simulink model "multi_sensor_with_filtering"  (R2018b)
settings: Solver=FixedStepAuto  StartTime=0.0  StopTime=inf  RelTol=1e-3  EnableMultiTasking=on
model workspace (MAT data in the model file):
  sensorControlMatrix = [0  0  0; 0  0  0; 0  0  0; 0  0  0; 0  0  0; 0  0  0; 1  0  0; 0  1  0; 0  0  1; 0  0  0; 0  0  0; 0  0  0; 0  0  0; 0  0  0; 0  0  0]
  sensorProcessNoiseMatrix = [1  0  0  0.02  0  0  0.0002  0  0  0  0  0  0  0  0; 0  1  0  0  0.02  0  0  0.0002  0  0  0  0  0  0  0; 0  0  1  0  0  0.02  0  0  0.0002  0  0  0  0  0  0; 0.02  0  0  1  0  0  0.02  0  0  0  0  0  0  0  0; 0  0.02  0  0  1  0  0  0.02  0  0  0  0  0  0  0; 0  0  0.02  0  0  1  0  0  0.02  0  0  0  0  0  0; 0.0002  0  0  0.02  0  0  1  0  0  0  0  0  0  0  0; 0  0.0002  0  0  0.02  0  0  1  0  0  0  0  0  0  0; 0  0  0.0002  0  0  0.02  0  0  1  0  0  0  0  0  0; 0  0  0  0  0  0  0  0  0  1  0  0  0.02  0  0; 0  0  0  0  0  0  0  0  0  0  1  0  0  0.02  0; 0  0  0  0  0  0  0  0  0  0  0  1  0  0  0.02; 0  0  0  0  0  0  0  0  0  0.02  0  0  1  0  0; 0  0  0  0  0  0  0  0  0  0  0.02  0  0  1  0; 0  0  0  0  0  0  0  0  0  0  0  0.02  0  0  1]
  sensorSampleTime = 0.01
  sensorSystemMatrix = [1  0  0  0.02  0  0  0.0002  0  0  0  0  0  0  0  0; 0  1  0  0  0.02  0  0  0.0002  0  0  0  0  0  0  0; 0  0  1  0  0  0.02  0  0  0.0002  0  0  0  0  0  0; 0  0  0  1  0  0  0.02  0  0  0  0  0  0  0  0; 0  0  0  0  1  0  0  0.02  0  0  0  0  0  0  0; 0  0  0  0  0  1  0  0  0.02  0  0  0  0  0  0; 0  0  0  0  0  0  1  0  0  0  0  0  0  0  0; 0  0  0  0  0  0  0  1  0  0  0  0  0  0  0; 0  0  0  0  0  0  0  0  1  0  0  0  0  0  0; 0  0  0  0  0  0  0  0  0  1  0  0  0.02  0  0; 0  0  0  0  0  0  0  0  0  0  1  0  0  0.02  0; 0  0  0  0  0  0  0  0  0  0  0  1  0  0  0.02; 0  0  0  0  0  0  0  0  0  0  0  0  1  0  0; 0  0  0  0  0  0  0  0  0  0  0  0  0  1  0; 0  0  0  0  0  0  0  0  0  0  0  0  0  0  1]
undefined symbols (not defined in the file): DiscIntNeverNeededParam, q
libraries: dspfdesign x5, sharedtransform x4, sharedTrackingLibrary x2, aerolibutil x2, simulink_extras x2, pil_lib x1
settings Model: SimulationMode=accelerator  ExtModeTrigDuration=2  Creator=Aliak  LastModifiedBy=Aliak
settings OptimizationCC: EnhancedBackFolding=on  PassReuseOutputArgsAs=Individual arguments  EfficientMapNaN2IntZero=off  MaxStackSize=64  OptimizeBlockOrder=speed  DifferentSizesBufferReuse=on  OptimizationCustomize=off
settings DebuggingCC: ParameterTunabilityLossMsg=error
settings HardwareCC: ProdBitPerInt=16  ProdBitPerPointer=16  ProdBitPerSizeT=16  ProdBitPerPtrDiffT=16  ProdWordSize=8  ProdHWDeviceType=Atmel->AVR  TargetBitPerPointer=64  TargetBitPerSizeT=64  TargetBitPerPtrDiffT=64  TargetLongLongMode=on  TargetIntDivRoundTo=Zero  TargetEndianess=LittleEndian  TargetWordSize=64  TargetHWDeviceType=MATLAB Host
settings SFSimCC: MATLABDynamicMemAlloc=off
settings RTWCC: SystemTargetFile=ert.tlc  HardwareBoard=Arduino Uno  TemplateMakefile=ert_default_tmf  GenerateReport=on  Toolchain=Arduino AVR  BuildConfiguration=Faster Runs  IncludeHyperlinkInReport=on  LaunchReport=on  CreateSILPILBlock=PIL  GenerateTraceInfo=on  GenerateTraceReport=on  GenerateTraceReportSl=on  GenerateTraceReportSf=on  GenerateTraceReportEml=on
settings CodeAppCC: ForceParamTrailComments=on  IgnoreCustomStorageClasses=off  MaxIdLength=128  OperatorAnnotations=on  SimulinkDataObjDesc=on  SFDataObjDesc=on  InsertBlockDesc=on
settings ERTTargetCC: SupportContinuousTime=on  SupportVariableSizeSignals=on

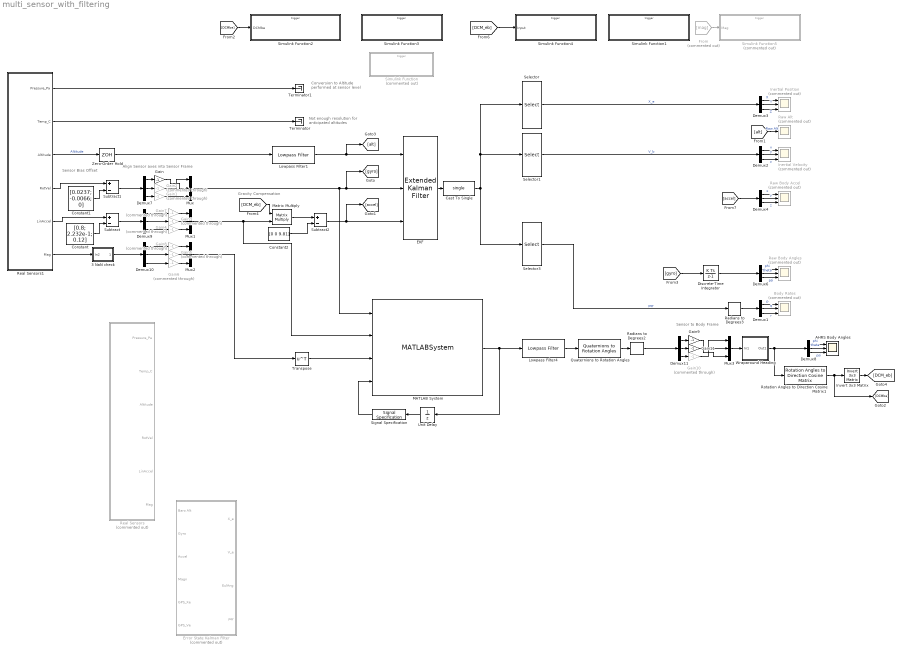
== system multi_sensor_with_filtering ==
  note: Sensor Bias Offset
  note: Gravity Compensation
  note: Align Sensor axes into Sensor Frame
  note: Sensor to Body Frame
  note: Conversion to Altitude performed at sensor level
  note: Not enough resolution for anticipated altitudes
  3 NaN check : Subsystem
  AHRS Body Angles : Scope  NumInputPorts=3
  Body Rates : Scope  Commented=on  NumInputPorts=3
  Cast To Single : DataTypeConversion  OutDataTypeStr=single
  Constant : Constant  Value=[0.8; 2.232e-1; 0.12]  VectorParams1D=off
  Constant1 : Constant  Value=[0.0237; -0.0066; 0]  VectorParams1D=off
  Constant2 : Constant  Value=[0 0 9.81]
  Demux{1..4,6..11} (10 alike) : Demux  Outputs=3
  Discrete-Time Integrator : DiscreteIntegrator  SampleTime=-1  ICPrevOutput=DiscIntNeverNeededParam  ICPrevScaledInput=DiscIntNeverNeededParam
  EKF : sharedTrackingLibrary/Extended Kalman Filter  StateTransitionFcn=sensorStateTransitionFcn  HasStateTransitionJacobianFcn=off  StateTransitionJacobianFcn=identityJacobianFcn  HasAdditiveProcessNoise=Additive  ProcessNoise=0.02  HasTimeVaryingProcessNoise=off  HasStateTransitionFcnExtraArgument=0  InitialState=single([0;0;49;0;0;0;0;0;0;0;0;0;0;0;0;])  InitialStateCovariance=0.0001  MeasurementFcn1=altMeasurementFcn  HasMeasurementJacobianFcn1=off  MeasurementJacobianFcn1=identityJacobianFcn  HasMeasurementEnablePort1=off  HasAdditiveMeasurementNoise1=Additive  MeasurementNoise1=0.18  HasTimeVaryingMeasurementNoise1=off  HasMeasurementFcnExtraArgument1=0  MeasurementFcn2=gyroMeasurementFcn  HasMeasurementJacobianFcn2=off  MeasurementJacobianFcn2=identityJacobianFcn  HasMeasurementEnablePort2=off  HasAdditiveMeasurementNoise2=Additive  MeasurementNoise2=0.1*eye(3)  HasTimeVaryingMeasurementNoise2=off  HasMeasurementFcnExtraArgument2=0  MeasurementFcn3=accelMeasurementFcn  HasMeasurementJacobianFcn3=off  MeasurementJacobianFcn3=identityJacobianFcn  HasMeasurementEnablePort3=off  HasAdditiveMeasurementNoise3=Additive  MeasurementNoise3=0.016*eye(3)  HasTimeVaryingMeasurementNoise3=off  HasMeasurementFcnExtraArgument3=0  MeasurementFcn4=magMeasurementFcn  HasMeasurementJacobianFcn4=off  MeasurementJacobianFcn4=identityJacobianFcn  HasMeasurementEnablePort4=off  HasAdditiveMeasurementNoise4=Additive  MeasurementNoise4=5*eye(3)  HasTimeVaryingMeasurementNoise4=off  HasMeasurementFcnExtraArgument4=0  MeasurementFcn5=myMeasurementFcn  HasMeasurementJacobianFcn5=off  HasMeasurementEnablePort5=off  HasAdditiveMeasurementNoise5=Additive  MeasurementNoise5=1  HasTimeVaryingMeasurementNoise5=off  HasMeasurementFcnExtraArgument5=0  EnableMultirate=off  StateTransitionFcnSampleTime=1  MeasurementFcn1SampleTime=1  MeasurementFcn2SampleTime=1  MeasurementFcn3SampleTime=1  MeasurementFcn4SampleTime=1  MeasurementFcn5SampleTime=1  UseCurrentEstimator=on  OutputStateCovariance=off  DataType=single  SampleTime=sensorSampleTime  NumberOfMeasurements=3
      settings: SourceProductName=Control System Toolbox  SourceProductBaseCode=CT
  Error State Kalman FIlter : Subsystem  Commented=on
  From : From  Commented=on  GotoTag=mag
  Gain : Gain  Gain=-1
  Gain{1..4,7,10} (6 alike) : Gain  Commented=through  Gain=-1
  Gain11 : Gain  Gain=-1
  Gain5 : Gain  Commented=through  Gain=-1  OutDataTypeStr=single
  Gain6 : Gain  Commented=through  Gain=-1  OutDataTypeStr=single
  Gain8 : Gain  Commented=through  Gain=-1  OutDataTypeStr=single
  Gain9 : Gain  Gain=-1
  Inertial Position : Scope  Commented=on  NumInputPorts=3
  Inertial Velocity : Scope  Commented=on  NumInputPorts=3
  Invert 3x3 Matrix : aerolibutil/Invert  3x3 Matrix
  Lowpass Filter1 : dspfdesign/Lowpass Filter  FilterType=IIR  DesignForMinimumOrder=on  FilterOrder=50  PassbandFrequency=250  StopbandFrequency=500  PassbandRipple=0.1  StopbandAttenuation=80  InheritSampleRate=off  SampleRate=1100  SimulateUsing=Code generation  roundingMode=Floor  coeffsDataTypeStr=fixdt(1,16)
  Lowpass Filter4 : dspfdesign/Lowpass Filter  FilterType=FIR  DesignForMinimumOrder=on  FilterOrder=50  PassbandFrequency=200  StopbandFrequency=300  PassbandRipple=0.1  StopbandAttenuation=80  InheritSampleRate=off  SampleRate=700  SimulateUsing=Code generation  roundingMode=Floor  coeffsDataTypeStr=fixdt(1,16)
  MATLAB System : MATLABSystem  System=MadgwickAHRSFilter  SamplePeriod=sensorSampleTime  Beta=5  SimulateUsing=Code generation
      mask Type: MadgwickAHRSFilter
      mask Display:
      | disp('MadgwickAHRSFilter');
      | port_label('input',1,'Gyroscope');
      | port_label('input',2,'Accelerometer');
      | port_label('input',3,'Magnetometer');
      | port_label('input',4,'q');
      | port_label('output',1,'quat');
  Matrix Multiply : Product  Multiplication=Matrix(*)
  Mux{,1..3} (4 alike) : Mux  Inputs=3
  Quaternions to Rotation Angles : sharedtransform/Quaternions to Rotation Angles  rotationOrder=ZYX  aMode=aMode
      settings: SourceProductBaseCode=AE
  Radians to Degrees2 : simulink_extras/Transformations/Radians to Degrees
  Radians to Degrees3 : simulink_extras/Transformations/Radians to Degrees
  Raw Alt : Scope  Commented=on
  Raw Body Accel : Scope  Commented=on  NumInputPorts=3
  Raw Body Angles : Scope  Commented=on  NumInputPorts=3
  Real Sensors : Subsystem  Commented=on  VariantControl=SimType==1
  Real Sensors1 : Subsystem  DialogController=pil_create_dialog  LoadFcn=|
      | try
      |    if ~strcmp(rtw.pil.getPILVersion, '9.5 (R2018b)_13')
      |       set_param(gcb, 'DialogController', '');
      |       set_param(gcb, 'DialogControllerArgs', '');
      |    end
      | catch e
      |       set_param(gcb, 'DialogController', '');
      |       set_param(gcb, 'DialogControllerArgs', '');
      | end
      mask help: PIL:pil:XILBlockMaskDesc
      mask Display: disp('PIL');
  Rotation Angles to Direction Cosine Matrix1 : sharedtransform/Rotation Angles to Direction Cosine Matrix  rotationOrder=XYZ  aMode=aMode
      settings: SourceProductBaseCode=AE
  Selector : Selector  IndexMode=Zero-based  InputPortWidth=15  IndexOptions=Index vector (dialog)  Indices=[0 1 2]  OutputSizes=1
  Selector1 : Selector  IndexMode=Zero-based  InputPortWidth=15  IndexOptions=Index vector (dialog)  Indices=[3 4 5]  OutputSizes=1
  Selector3 : Selector  IndexMode=Zero-based  InputPortWidth=15  IndexOptions=Index vector (dialog)  Indices=[12 13 14]  OutputSizes=1
  Signal Specification : SignalSpecification  OutDataTypeStr=single  Dimensions=[1 4]
  Simulink Function : Subsystem  Commented=on  TreatAsAtomicUnit=on
  Simulink Function1 : Subsystem  TreatAsAtomicUnit=on
  Simulink Function2 : Subsystem  TreatAsAtomicUnit=on
  Simulink Function3 : Subsystem  TreatAsAtomicUnit=on
  Simulink Function4 : Subsystem  TreatAsAtomicUnit=on
  Simulink Function5 : Subsystem  Commented=on  TreatAsAtomicUnit=on
  Subtract : Sum  Inputs=+-  OutDataTypeStr=single
  Subtract1 : Sum  Inputs=+-  OutDataTypeStr=single
  Subtract2 : Sum  Inputs=+-  OutDataTypeStr=single
  Terminator : Terminator
  Terminator1 : Terminator
  Transpose : Math  Operator=transpose  SaturateOnIntegerOverflow=on
  Unit Delay : UnitDelay  InitialCondition=[1 0 0 0]  SampleTime=sensorSampleTime
  Wraparound Heading : Subsystem
  Zero-Order Hold : ZeroOrderHold  SampleTime=sensorSampleTime
  wires:
  Selector3/1 -> Radians to Degrees3/1  "pqr"
  Cast To Single/1 -> Selector/1, Selector1/1, Selector3/1
  From/1 -> Simulink Function5/1(Mag)
  Subtract/1 -> Demux9/1
  EKF/1 -> Cast To Single/1
  [DCMbe] -> Simulink Function2/1(DCMbe)
  Selector/1 -> Demux3/1  "X_e"
  Selector1/1 -> Demux2/1  "V_b"
  Radians to Degrees3/1 -> Demux1/1
  Demux1/1 -> Body Rates/1  "p"
  Demux1/2 -> Body Rates/2  "q"
  Demux1/3 -> Body Rates/3  "r"
  Demux2/1 -> Inertial Velocity/1  "x"
  Demux2/2 -> Inertial Velocity/2  "y"
  Demux2/3 -> Inertial Velocity/3  "z"
  Demux3/1 -> Inertial Position/1  "X"
  Demux3/2 -> Inertial Position/2  "Y"
  Demux3/3 -> Inertial Position/3  "Z"
  [accel] -> Demux4/1
  Demux4/2 -> Raw Body Accel/2  "y"
  Demux4/1 -> Raw Body Accel/1  "x"
  Demux4/3 -> Raw Body Accel/3  "z"
  Constant/1 -> Subtract/2
  Constant1/1 -> Subtract1/2
  [alt] -> Raw Alt/1  "Raw Alt"
  Demux6/3 -> Raw Body Angles/3  "psi"
  Demux6/1 -> Raw Body Angles/1  "phi"
  Demux6/2 -> Raw Body Angles/2  "theta"
  [gyro] -> Discrete-Time Integrator/1
  Discrete-Time Integrator/1 -> Demux6/1
  Subtract1/1 -> Demux7/1
  Demux8/3 -> AHRS Body Angles/3  "psi"
  Demux8/2 -> AHRS Body Angles/2  "theta"
  Quaternions to Rotation Angles/1 -> Radians to Degrees2/1
  Demux8/1 -> AHRS Body Angles/1  "phi"
  Transpose/1 -> MATLAB System/3
  Lowpass Filter1/1 -> EKF/1, [alt]
  Mux/1 -> EKF/2, [gyro], MATLAB System/1
  Zero-Order Hold/1 -> Lowpass Filter1/1
  Real Sensors1/2(Temp_C) -> Terminator/1
  Real Sensors1/3(Altitude) -> Zero-Order Hold/1  "Altitude"
  Real Sensors1/5(LinAccel) -> Subtract/1
  Real Sensors1/1(Pressure_Pa) -> Terminator1/1
  Mux2/1 -> Transpose/1
  Real Sensors1/4(RotVel) -> Subtract1/1
  [DCM_eb] -> Matrix Multiply/1
  Subtract2/1 -> [accel], EKF/3
  [DCM_eb] -> Simulink Function4/1(Input)
  Invert 3x3 Matrix/1 -> [DCM_eb]
  Rotation Angles to Direction Cosine Matrix1/1 -> [DCMbe], Invert 3x3 Matrix/1
  Matrix Multiply/1 -> Subtract2/1
  Constant2/1 -> Subtract2/2
  Unit Delay/1 -> Signal Specification/1
  MATLAB System/1 -> Lowpass Filter4/1, Unit Delay/1
  Signal Specification/1 -> MATLAB System/4
  Mux1/1 -> MATLAB System/2, Matrix Multiply/2
  Real Sensors1/6(Mag) -> 3 NaN check/1(In2)
  3 NaN check/1(Out1) -> Demux10/1
  Lowpass Filter4/1 -> Quaternions to Rotation Angles/1
  Demux10/3 -> Gain6/1
  Demux10/1 -> Gain8/1
  Demux10/2 -> Gain5/1
  Demux9/3 -> Gain4/1
  Demux9/2 -> Gain3/1
  Demux9/1 -> Gain7/1
  Demux7/3 -> Gain1/1
  Demux7/1 -> Gain/1
  Demux7/2 -> Gain2/1
  Gain3/1 -> Mux1/2
  Gain4/1 -> Mux1/3
  Gain5/1 -> Mux2/2
  Gain6/1 -> Mux2/3
  Gain7/1 -> Mux1/1
  Gain8/1 -> Mux2/1
  Gain2/1 -> Mux/1
  Gain/1 -> Mux/2
  Gain1/1 -> Mux/3
  Wraparound Heading/1(Out1) -> Demux8/1, Rotation Angles to Direction Cosine Matrix1/1
  Radians to Degrees2/1 -> Demux11/1
  Demux11/3 -> Gain10/1
  Demux11/2 -> Gain11/1
  Gain9/1 -> Mux3/3
  Gain11/1 -> Mux3/2
  Gain10/1 -> Mux3/1
  Demux11/1 -> Gain9/1
  Mux3/1 -> Wraparound Heading/1(In1)

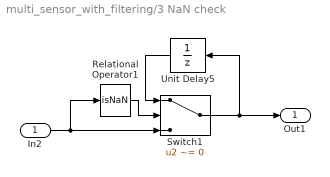
== system multi_sensor_with_filtering/3 NaN check ==
  In2 : Inport
  Relational Operator1 : RelationalOperator  Operator=isNaN  OutDataTypeStr=boolean  RndMeth=Simplest
  Switch1 : Switch  Criteria=u2 ~= 0
  Unit Delay5 : UnitDelay  InitialCondition=[0; 0; 0]  SampleTime=-1
  Out1 : Outport
  wires:
  Relational Operator1/1 -> Switch1/2
  Unit Delay5/1 -> Switch1/1
  Switch1/1 -> Unit Delay5/1, Out1/1
  In2/1 -> Relational Operator1/1, Switch1/3

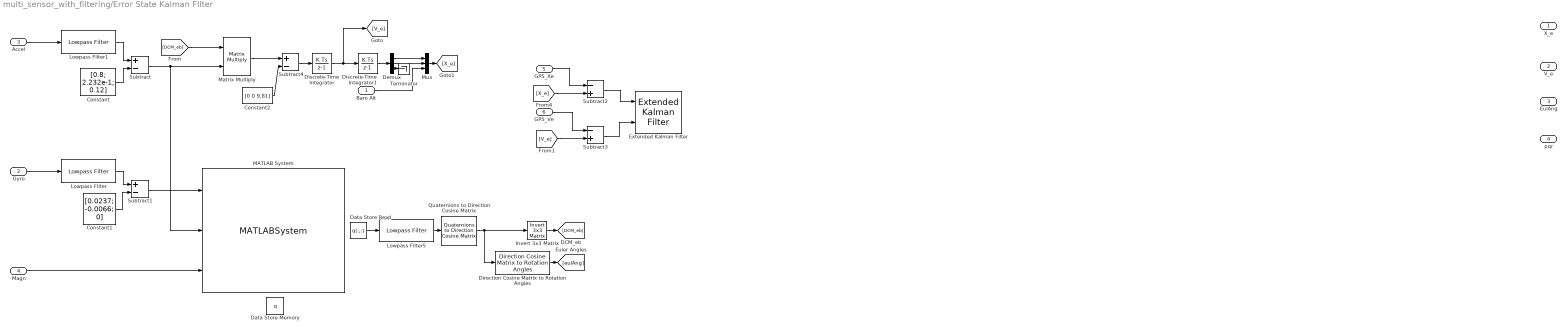
== system multi_sensor_with_filtering/Error State Kalman FIlter ==
  Baro Alt : Inport
  Gyro : Inport  Port=2
  Accel : Inport  Port=3
  Magn : Inport  Port=4
  GPS_Xe : Inport  Port=5
  GPS_Ve : Inport  Port=6
  Constant : Constant  Value=[0.8; 2.232e-1; 0.12]  VectorParams1D=off
  Constant1 : Constant  Value=[0.0237; -0.0066; 0]  VectorParams1D=off
  Constant2 : Constant  Value=[0 0 9.81]  VectorParams1D=off
  Data Store Memory : DataStoreMemory  DataStoreName=q  ReadBeforeWriteMsg=warning  WriteAfterWriteMsg=warning  WriteAfterReadMsg=warning  InitialValue=[1 0 0 0]  VectorParams1D=off  ShowAdditionalParam=off  OutDataTypeStr=single  Dimensions=[1 4]
  Data Store Read : DataStoreRead  DataStoreName=q  DataStoreElements=q(:,:)
  Demux : Demux  Outputs=3
  Direction Cosine Matrix to Rotation Angles : sharedtransform/Direction Cosine Matrix to Rotation Angles  rotationOrder=ZYX  aMode=aMode  action=None  tolerance=eps(2)
      settings: SourceProductName=Aerospace Blockset  SourceProductBaseCode=AE
  Discrete-Time Integrator : DiscreteIntegrator  SampleTime=-1  ICPrevOutput=DiscIntNeverNeededParam  ICPrevScaledInput=DiscIntNeverNeededParam
  Discrete-Time Integrator1 : DiscreteIntegrator  SampleTime=-1  ICPrevOutput=DiscIntNeverNeededParam  ICPrevScaledInput=DiscIntNeverNeededParam
  Extended Kalman Filter : sharedTrackingLibrary/Extended Kalman Filter  StateTransitionFcn=myStateTransitionFcn  HasStateTransitionJacobianFcn=off  HasAdditiveProcessNoise=Additive  ProcessNoise=1  HasTimeVaryingProcessNoise=off  HasStateTransitionFcnExtraArgument=0  InitialState=0  InitialStateCovariance=1  MeasurementFcn1=myMeasurementFcn  HasMeasurementJacobianFcn1=off  HasMeasurementEnablePort1=off  HasAdditiveMeasurementNoise1=Additive  MeasurementNoise1=1  HasTimeVaryingMeasurementNoise1=off  HasMeasurementFcnExtraArgument1=0  MeasurementFcn2=myMeasurementFcn  HasMeasurementJacobianFcn2=off  HasMeasurementEnablePort2=off  HasAdditiveMeasurementNoise2=Additive  MeasurementNoise2=1  HasTimeVaryingMeasurementNoise2=off  HasMeasurementFcnExtraArgument2=0  MeasurementFcn3=myMeasurementFcn  HasMeasurementJacobianFcn3=off  HasMeasurementEnablePort3=off  HasAdditiveMeasurementNoise3=Additive  MeasurementNoise3=1  HasTimeVaryingMeasurementNoise3=off  HasMeasurementFcnExtraArgument3=0  MeasurementFcn4=myMeasurementFcn  HasMeasurementJacobianFcn4=off  HasMeasurementEnablePort4=off  HasAdditiveMeasurementNoise4=Additive  MeasurementNoise4=1  HasTimeVaryingMeasurementNoise4=off  HasMeasurementFcnExtraArgument4=0  MeasurementFcn5=myMeasurementFcn  HasMeasurementJacobianFcn5=off  HasMeasurementEnablePort5=off  HasAdditiveMeasurementNoise5=Additive  MeasurementNoise5=1  HasTimeVaryingMeasurementNoise5=off  HasMeasurementFcnExtraArgument5=0  EnableMultirate=off  StateTransitionFcnSampleTime=1  MeasurementFcn1SampleTime=1  MeasurementFcn2SampleTime=1  MeasurementFcn3SampleTime=1  MeasurementFcn4SampleTime=1  MeasurementFcn5SampleTime=1  UseCurrentEstimator=on  OutputStateCovariance=off  DataType=single  SampleTime=sensorSampleTime  NumberOfMeasurements=2
      settings: SourceProductName=Control System Toolbox  SourceProductBaseCode=CT
  Invert 3x3 Matrix : aerolibutil/Invert  3x3 Matrix
  Lowpass Filter : dspfdesign/Lowpass Filter  FilterType=FIR  DesignForMinimumOrder=on  FilterOrder=50  PassbandFrequency=8e3  StopbandFrequency=12e3  PassbandRipple=0.1  StopbandAttenuation=80  InheritSampleRate=off  SampleRate=44100  SimulateUsing=Interpreted execution  roundingMode=Floor  coeffsDataTypeStr=fixdt(1,16)
  Lowpass Filter1 : dspfdesign/Lowpass Filter  FilterType=FIR  DesignForMinimumOrder=on  FilterOrder=50  PassbandFrequency=8e3  StopbandFrequency=12e3  PassbandRipple=0.1  StopbandAttenuation=80  InheritSampleRate=off  SampleRate=44100  SimulateUsing=Interpreted execution  roundingMode=Floor  coeffsDataTypeStr=fixdt(1,16)
  Lowpass Filter5 : dspfdesign/Lowpass Filter  FilterType=FIR  DesignForMinimumOrder=on  FilterOrder=50  PassbandFrequency=500  StopbandFrequency=1000  PassbandRipple=0.1  StopbandAttenuation=80  InheritSampleRate=off  SampleRate=5000  SimulateUsing=Code generation  roundingMode=Floor  coeffsDataTypeStr=fixdt(1,16)
  MATLAB System : MATLABSystem  System=MadgwickAHRSFilter  SamplePeriod=sensorSampleTime  Beta=30  SimulateUsing=Code generation
      mask Type: MadgwickAHRSFilter
      mask Display:
      | disp('MadgwickAHRSFilter');
      | port_label('input',1,'Gyroscope');
      | port_label('input',2,'Accelerometer');
      | port_label('input',3,'Magnetometer');
  Matrix Multiply : Product  Multiplication=Matrix(*)
  Mux : Mux  Inputs=3
  Quaternions to Direction Cosine Matrix : sharedtransform/Quaternions to  Direction Cosine Matrix  aMode=aMode
      settings: SourceProductName=Aerospace Blockset  SourceProductBaseCode=AE
  Subtract : Sum  Inputs=+-  OutDataTypeStr=single
  Subtract1 : Sum  Inputs=+-  OutDataTypeStr=single
  Subtract2 : Sum  Inputs=-+
  Subtract3 : Sum  Inputs=-+
  Subtract4 : Sum  Inputs=+-
  Terminator : Terminator
  X_e : Outport
  V_e : Outport  Port=2
  EulAng : Outport  Port=3
  pqr : Outport  Port=4
  wires:
  Gyro/1 -> Lowpass Filter/1
  Accel/1 -> Lowpass Filter1/1
  Constant/1 -> Subtract/2
  Lowpass Filter1/1 -> Subtract/1
  Constant1/1 -> Subtract1/2
  Lowpass Filter/1 -> Subtract1/1
  Subtract1/1 -> MATLAB System/1
  Subtract/1 -> Matrix Multiply/2, MATLAB System/2
  Magn/1 -> MATLAB System/3
  Data Store Read/1 -> Lowpass Filter5/1
  Lowpass Filter5/1 -> Quaternions to Direction Cosine Matrix/1
  Quaternions to Direction Cosine Matrix/1 -> Direction Cosine Matrix to Rotation Angles/1, Invert 3x3 Matrix/1
  Invert 3x3 Matrix/1 -> [DCM_eb]
  [DCM_eb] -> Matrix Multiply/1
  Matrix Multiply/1 -> Subtract4/1
  Discrete-Time Integrator/1 -> [V_e], Discrete-Time Integrator1/1
  [V_e] -> Subtract3/2
  Direction Cosine Matrix to Rotation Angles/1 -> [eulAng]
  Discrete-Time Integrator1/1 -> Demux/1
  [X_e] -> Subtract2/2
  Mux/1 -> [X_e]
  Demux/1 -> Mux/1
  Demux/2 -> Mux/2
  Baro Alt/1 -> Mux/3
  Demux/3 -> Terminator/1
  GPS_Xe/1 -> Subtract2/1
  GPS_Ve/1 -> Subtract3/1
  Subtract2/1 -> Extended Kalman Filter/1
  Subtract3/1 -> Extended Kalman Filter/2
  Subtract4/1 -> Discrete-Time Integrator/1
  Constant2/1 -> Subtract4/2

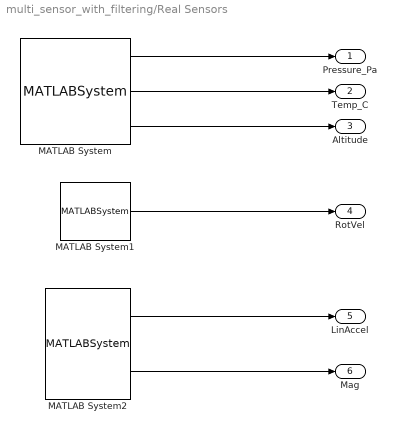
== system multi_sensor_with_filtering/Real Sensors ==
  MATLAB System : MATLABSystem  System=BMP085  Reference_Pressure=101200  SimulateUsing=Code generation
      mask Type: BMP085
      mask Display:
      | disp('BMP085');
      | port_label('output',1,'press');
      | port_label('output',2,'temp');
      | port_label('output',3,'alt');
  MATLAB System1 : MATLABSystem  System=L3GD20  SimulateUsing=Code generation
      mask Type: L3GD20
      mask Display:
      | disp('L3GD20');
      | port_label('output',1,'rot');
  MATLAB System2 : MATLABSystem  System=LSM303  SimulateUsing=Code generation
      mask Type: LSM303
      mask Display:
      | disp('LSM303');
      | port_label('output',1,'accel');
      | port_label('output',2,'mag');
  Pressure_Pa : Outport
  Temp_C : Outport  Port=2
  Altitude : Outport  Port=3
  RotVel : Outport  Port=4
  LinAccel : Outport  Port=5
  Mag : Outport  Port=6
  wires:
  MATLAB System/1 -> Pressure_Pa/1
  MATLAB System/2 -> Temp_C/1
  MATLAB System/3 -> Altitude/1
  MATLAB System1/1 -> RotVel/1
  MATLAB System2/1 -> LinAccel/1
  MATLAB System2/2 -> Mag/1

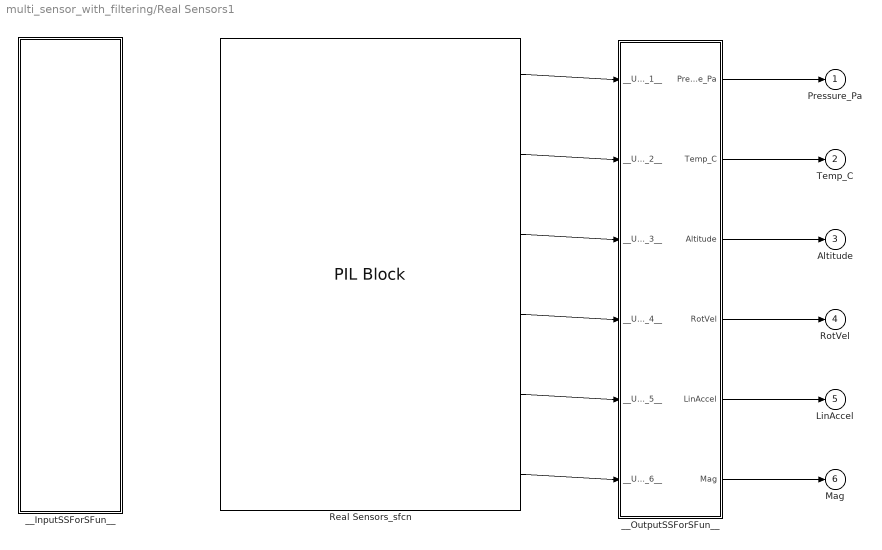
== system multi_sensor_with_filtering/Real Sensors1 ==
  Real Sensors_sfcn : pil_lib/PIL Block  SimulationMode=PIL  IsTopModelPIL=off  CodeDir=D:\MATLABProjects\FEEG2001-FWUAV\tests\Real0_ert_rtw  AnchorDir=D:\MATLABProjects\FEEG2001-FWUAV\tests  ConfigName=Arduino Board  XrelIsTopModelCode=on  XrelIsReusable=off  XrelDWorkNames={}  XrelDWorkTypes={}  XrelModelArgVals={}  XrelOrderedParamNames={}
  __InputSSForSFun__ : Subsystem
  __OutputSSForSFun__ : Subsystem
  Pressure_Pa : Outport
  Temp_C : Outport  Port=2
  Altitude : Outport  Port=3
  RotVel : Outport  Port=4
  LinAccel : Outport  Port=5
  Mag : Outport  Port=6
  wires:
  Real Sensors_sfcn/1 -> __OutputSSForSFun__/1(__UniqueInportName__1__)
  Real Sensors_sfcn/2 -> __OutputSSForSFun__/2(__UniqueInportName__2__)
  Real Sensors_sfcn/3 -> __OutputSSForSFun__/3(__UniqueInportName__3__)
  Real Sensors_sfcn/4 -> __OutputSSForSFun__/4(__UniqueInportName__4__)
  Real Sensors_sfcn/5 -> __OutputSSForSFun__/5(__UniqueInportName__5__)
  Real Sensors_sfcn/6 -> __OutputSSForSFun__/6(__UniqueInportName__6__)
  __OutputSSForSFun__/1(Pressure_Pa) -> Pressure_Pa/1
  __OutputSSForSFun__/2(Temp_C) -> Temp_C/1
  __OutputSSForSFun__/3(Altitude) -> Altitude/1
  __OutputSSForSFun__/4(RotVel) -> RotVel/1
  __OutputSSForSFun__/5(LinAccel) -> LinAccel/1
  __OutputSSForSFun__/6(Mag) -> Mag/1

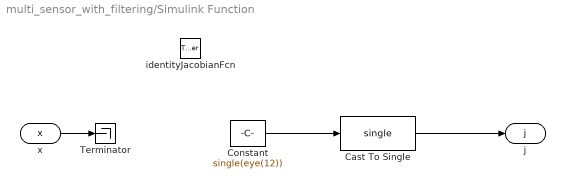
== system multi_sensor_with_filtering/Simulink Function ==
  identityJacobianFcn : TriggerPort  TriggerType=function-call  IsSimulinkFunction=on  FunctionName=identityJacobianFcn  FunctionVisibility=scoped  VariantControl=(inherit)
  Cast To Single : DataTypeConversion  OutDataTypeStr=single
  Constant : Constant  Value=single(eye(12))
  Terminator : Terminator
  x : ArgIn  DisableCoverage=on  OutDataTypeStr=single  PortDimensions=12  ArgumentName=x
  j : ArgOut  DisableCoverage=on  OutDataTypeStr=single  PortDimensions=[12 12]  ArgumentName=j
  wires:
  x/1 -> Terminator/1
  Constant/1 -> Cast To Single/1
  Cast To Single/1 -> j/1

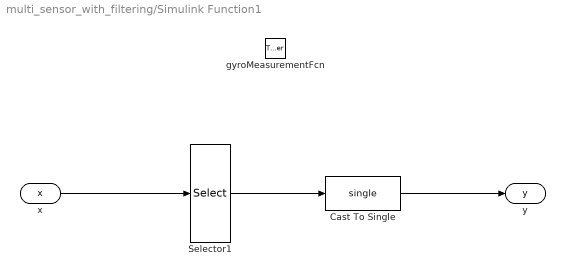
== system multi_sensor_with_filtering/Simulink Function1 ==
  gyroMeasurementFcn : TriggerPort  TriggerType=function-call  IsSimulinkFunction=on  FunctionName=gyroMeasurementFcn  FunctionVisibility=scoped  VariantControl=(inherit)
  Cast To Single : DataTypeConversion  OutDataTypeStr=single
  Selector1 : Selector  IndexMode=Zero-based  InputPortWidth=15  IndexOptions=Index vector (dialog)  Indices=[12 13 14]  OutputSizes=1
  x : ArgIn  OutDataTypeStr=single  PortDimensions=15  ArgumentName=x
  y : ArgOut  DisableCoverage=on  OutDataTypeStr=single  PortDimensions=3  ArgumentName=y
  wires:
  Selector1/1 -> Cast To Single/1
  x/1 -> Selector1/1
  Cast To Single/1 -> y/1

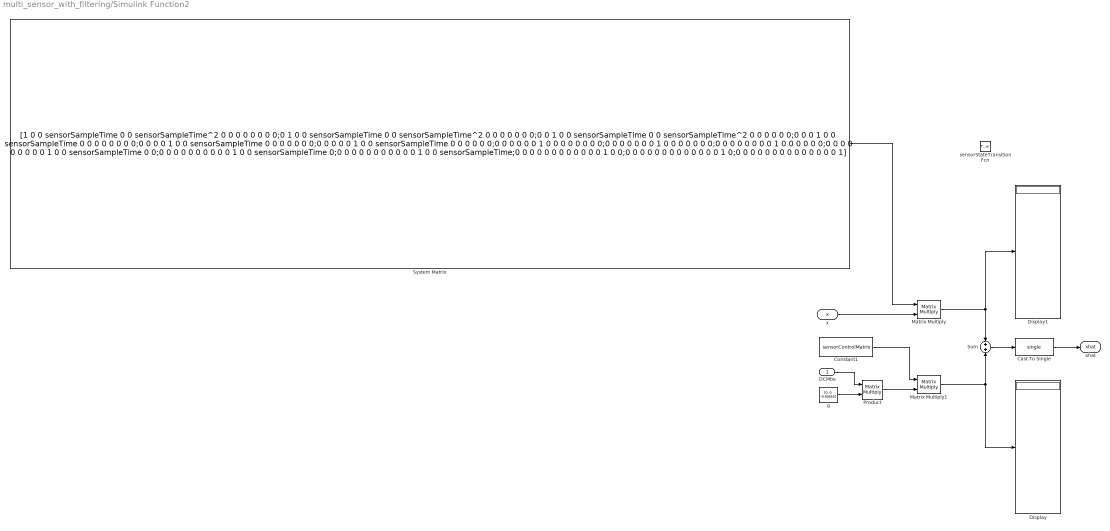
== system multi_sensor_with_filtering/Simulink Function2 ==
  DCMbe : Inport
  sensorStateTransitionFcn : TriggerPort  TriggerType=function-call  IsSimulinkFunction=on  FunctionName=sensorStateTransitionFcn  FunctionVisibility=scoped  VariantControl=(inherit)
  Cast To Single : DataTypeConversion  OutDataTypeStr=single
  Constant1 : Constant  Value=sensorControlMatrix  VectorParams1D=off
  Display : Display
      settings: Decimation=3
  Display1 : Display
      settings: Decimation=3
  Matrix Multiply : Product  Multiplication=Matrix(*)
  Matrix Multiply1 : Product  Multiplication=Matrix(*)
  Product : Product  Multiplication=Matrix(*)
  Sum : Sum
  System Matrix : Constant  Value=[1 0 0 sensorSampleTime 0 0 sensorSampleTime^2 0 0 0 0 0 0 0 0;0 1 0 0 sensorSampleTime 0 0 sensorSampleTime^2 0 0 0 0 0 0 0;0 0 1 0 0 sensorSampleTime 0 0 sensorSampleTime^2 0 0 0 0 0 0;0 0 0 1 0 0 sensorSampleTime 0 0 0 0 0 0 0 0;0 0 0 0 1 0 0 sensorSampleTime 0 0 0 0 0 0 0;0 0 0 0 0 1 0 0 sensorSampleTime 0 0 0 0 0 0;0 0 0 0 0 0 1 0 0 0 0 0 0 0 0;0 0 0 0 0 0 0 1 0 0 0 0 0 0 0;0 0 0 0 0 0 0 0 1 0 0 0 0 0 0;0 0 0 0 0 0 0 0 0 1 0 0 sensorSampleTime 0 0;0 0 0 0 0 0 0 0 0 0 1 0 0 sensorSampleTime 0;0 0 0 0 0 0 0 0 0 0 0 1 0 0 sensorSampleTime;0 0 0 0 0 0 0 0 0 0 0 0 1 0 0;0 0 0 0 0 0 0 0 0 0 0 0 0 1 0;0 0 0 0 0 0 0 0 0 0 0 0 0 0 1]  VectorParams1D=off
  g : Constant  Value=[0; 0; -9.80665]  VectorParams1D=off
  x : ArgIn  DisableCoverage=on  OutDataTypeStr=single  PortDimensions=15  ArgumentName=x
  xhat : ArgOut  DisableCoverage=on  OutDataTypeStr=single  PortDimensions=15  ArgumentName=xhat
  wires:
  x/1 -> Matrix Multiply/2
  System Matrix/1 -> Matrix Multiply/1
  Matrix Multiply/1 -> Display1/1, Sum/1
  DCMbe/1 -> Product/1
  Sum/1 -> Cast To Single/1
  g/1 -> Product/2
  Cast To Single/1 -> xhat/1
  Product/1 -> Matrix Multiply1/2
  Matrix Multiply1/1 -> Sum/2, Display/1
  Constant1/1 -> Matrix Multiply1/1

== system multi_sensor_with_filtering/Simulink Function3 ==
  altMeasurementFcn : TriggerPort  TriggerType=function-call  IsSimulinkFunction=on  FunctionName=altMeasurementFcn  FunctionVisibility=scoped  VariantControl=(inherit)
  Cast To Single : DataTypeConversion  OutDataTypeStr=single
  Selector : Selector  IndexMode=Zero-based  InputPortWidth=15  IndexOptions=Index vector (dialog)  Indices=2  OutputSizes=1
  x : ArgIn  DisableCoverage=on  OutDataTypeStr=single  PortDimensions=15  ArgumentName=x
  y : ArgOut  DisableCoverage=on  OutDataTypeStr=single  ArgumentName=y
  wires:
  x/1 -> Selector/1
  Selector/1 -> Cast To Single/1
  Cast To Single/1 -> y/1

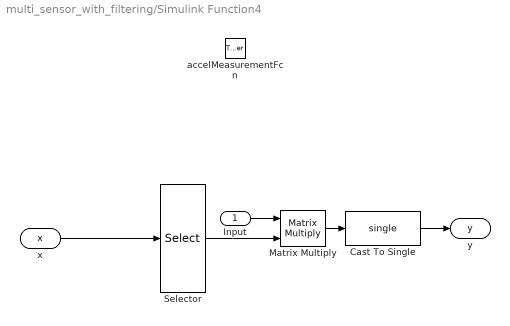
== system multi_sensor_with_filtering/Simulink Function4 ==
  Input : Inport
  accelMeasurementFcn : TriggerPort  TriggerType=function-call  IsSimulinkFunction=on  FunctionName=accelMeasurementFcn  FunctionVisibility=scoped  VariantControl=(inherit)
  Cast To Single : DataTypeConversion  OutMin=-100  OutMax=100  OutDataTypeStr=single
  Matrix Multiply : Product  Multiplication=Matrix(*)
  Selector : Selector  IndexMode=Zero-based  InputPortWidth=15  IndexOptions=Index vector (dialog)  Indices=[6 7 8]  OutputSizes=1
  x : ArgIn  DisableCoverage=on  OutDataTypeStr=single  PortDimensions=15  ArgumentName=x
  y : ArgOut  DisableCoverage=on  OutDataTypeStr=single  PortDimensions=3  ArgumentName=y
  wires:
  x/1 -> Selector/1
  Selector/1 -> Matrix Multiply/2
  Cast To Single/1 -> y/1
  Matrix Multiply/1 -> Cast To Single/1
  Input/1 -> Matrix Multiply/1

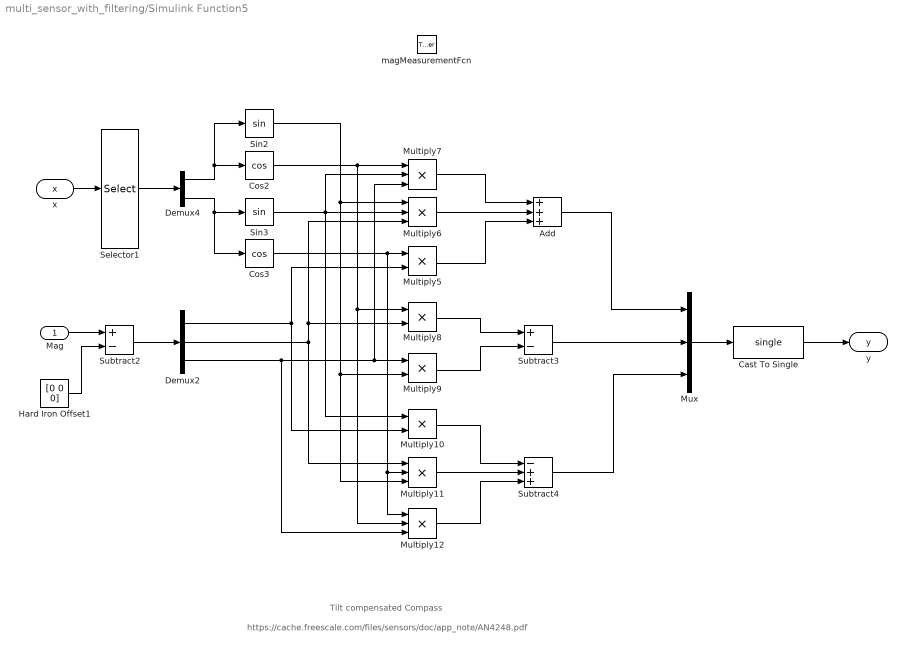
== system multi_sensor_with_filtering/Simulink Function5 ==
  note: https://cache.freescale.com/files/sensors/doc/app_note/AN4248.pdf
  note: Tilt compensated Compass
  Mag : Inport
  magMeasurementFcn : TriggerPort  TriggerType=function-call  IsSimulinkFunction=on  FunctionName=magMeasurementFcn  FunctionVisibility=scoped  VariantControl=(inherit)
  Add : Sum  Inputs=+++
  Cast To Single : DataTypeConversion  OutDataTypeStr=single
  Cos2 : Trigonometry  Operator=cos
  Cos3 : Trigonometry  Operator=cos
  Demux2 : Demux  Outputs=3
  Demux4 : Demux  Outputs=2
  Hard Iron Offset1 : Constant  Value=[0 0 0]
  Multiply{5,8..10} (4 alike) : Product
  Multiply{6..7,11..12} (4 alike) : Product  Inputs=3
  Mux : Mux  Inputs=3
  Selector1 : Selector  IndexMode=Zero-based  InputPortWidth=15  IndexOptions=Index vector (dialog)  Indices=[9 10]  OutputSizes=1
  Sin2 : Trigonometry
  Sin3 : Trigonometry
  Subtract2 : Sum  Inputs=+-
  Subtract3 : Sum  Inputs=+-
  Subtract4 : Sum  Inputs=-++
  x : ArgIn  OutDataTypeStr=single  PortDimensions=15  ArgumentName=x
  y : ArgOut  DisableCoverage=on  OutDataTypeStr=single  PortDimensions=3  ArgumentName=y
  wires:
  x/1 -> Selector1/1
  Mux/1 -> Cast To Single/1
  Hard Iron Offset1/1 -> Subtract2/2
  Subtract2/1 -> Demux2/1
  Demux4/1 -> Sin2/1, Cos2/1
  Demux4/2 -> Cos3/1, Sin3/1
  Selector1/1 -> Demux4/1
  Cos3/1 -> Multiply12/1, Multiply11/2, Multiply5/1
  Demux2/1 -> Multiply10/2, Multiply5/2
  Demux2/2 -> Multiply11/1, Multiply6/3, Multiply8/2
  Sin3/1 -> Multiply6/2, Multiply10/1, Multiply7/2
  Sin2/1 -> Multiply6/1, Multiply11/3, Multiply9/2
  Cos2/1 -> Multiply12/2, Multiply8/1, Multiply7/1
  Demux2/3 -> Multiply12/3, Multiply9/1, Multiply7/3
  Multiply7/1 -> Add/1
  Multiply6/1 -> Add/2
  Multiply5/1 -> Add/3
  Add/1 -> Mux/1
  Multiply8/1 -> Subtract3/1
  Multiply9/1 -> Subtract3/2
  Subtract3/1 -> Mux/2
  Multiply10/1 -> Subtract4/1
  Multiply11/1 -> Subtract4/2
  Multiply12/1 -> Subtract4/3
  Subtract4/1 -> Mux/3
  Cast To Single/1 -> y/1
  Mag/1 -> Subtract2/1

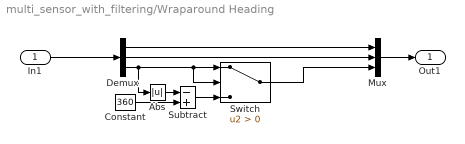
== system multi_sensor_with_filtering/Wraparound Heading ==
  In1 : Inport
  Abs : Abs
  Constant : Constant  Value=360
  Demux : Demux  Outputs=3
  Mux : Mux  Inputs=3
  Subtract : Sum  Inputs=-+
  Switch : Switch  Criteria=u2 > Threshold  OutDataTypeStr=single
  Out1 : Outport
  wires:
  In1/1 -> Demux/1
  Mux/1 -> Out1/1
  Demux/1 -> Mux/1
  Demux/2 -> Mux/2
  Demux/3 -> Abs/1, Switch/2, Switch/1
  Switch/1 -> Mux/3
  Subtract/1 -> Switch/3
  Constant/1 -> Subtract/2
  Abs/1 -> Subtract/1

== system multi_sensor_with_filtering/Real Sensors1/__InputSSForSFun__ ==

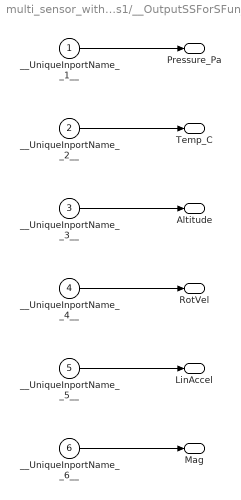
== system multi_sensor_with_filtering/Real Sensors1/__OutputSSForSFun__ ==
  __UniqueInportName__1__ : Inport
  __UniqueInportName__2__ : Inport  Port=2
  __UniqueInportName__3__ : Inport  Port=3
  __UniqueInportName__4__ : Inport  Port=4
  __UniqueInportName__5__ : Inport  Port=5
  __UniqueInportName__6__ : Inport  Port=6
  Pressure_Pa : Outport
  Temp_C : Outport  Port=2
  Altitude : Outport  Port=3
  RotVel : Outport  Port=4
  LinAccel : Outport  Port=5
  Mag : Outport  Port=6
  wires:
  __UniqueInportName__1__/1 -> Pressure_Pa/1
  __UniqueInportName__2__/1 -> Temp_C/1
  __UniqueInportName__3__/1 -> Altitude/1
  __UniqueInportName__4__/1 -> RotVel/1
  __UniqueInportName__5__/1 -> LinAccel/1
  __UniqueInportName__6__/1 -> Mag/1
